simulink model "non_lin_dyn_model"  (R2024b)
settings: Solver=ode4  StartTime=0.0  StopTime=30  FixedStep=ST  RelTol=1e-3
values from neighbouring files (symbols this model uses):
  AOP = 2.75*pi/180    (= 0.0479965544298)    [parameters.m]
  AOPTR = 0    [parameters.m]
  ASLOPE = 6.28    [parameters.m]
  ASLOPETR = 6.28    [parameters.m]
  att_sp = 0    [FEL_RBFNN.m]    (also in results.m)
  Ax = 5.5*0.3048^2    (= 0.51096672)    [parameters.m]
  Ay = 156.1*0.3048^2    (= 14.502164544)    [parameters.m]
  Az = 84.7*0.3048^2    (= 7.868887488)    [parameters.m]
  B_inv = inv(B*B_dim)    [parameters.m]
  BLADES = 2    [parameters.m]
  BLADESTR = 2    [parameters.m]
  CD_mr = [0.009 0 0.3]    [parameters.m]
  CD_tr = [0.009 0 0.3]    [parameters.m]
  CHORD = 2.25*Ft_m    (= 0.6858)    [parameters.m]
  CHORDTR = 0.7*Ft_m    (= 0.21336)    [parameters.m]
  eta = 1    [FEL_RBFNN.m]
  f = [ 0; 0; Q_mr_trim/Izz]    [parameters.m]
  g = 9.81    [parameters.m]
  GAMMA = 5.216    [parameters.m]
  k = diag([3.7,5,10])    [FEL_RBFNN.m]
  k_ind = 1    [parameters.m]
  L_fus = [ -0.1 ... (first row only)    [parameters.m]
  L_mr = [  -0.1 ... (first row only)    [parameters.m]
  L_tr = [  -8.25 ... (first row only)    [parameters.m]
  lambda = diag([0.08,0.05,1.5])    [FEL_RBFNN.m]
  lat_cyc_range = [ -15 15 ]    [parameters.m]
  lon_cyc_range = [ -15 15 ]    [parameters.m]
  m = 8000*Lb_Kg    (= 3628.736)    [parameters.m]
  mr_coll_range = [ 7.5 25 ]    [parameters.m]
  NN_state = 1    [FEL_RBFNN.m]    (also in results.m)
  OMEGA = 314*(pi/30)    (= 32.8820031076)    [parameters.m]
  OMEGATR = 1608.5*(pi/30)    (= 168.44172611)    [parameters.m]
  pilot_trim = [-0.11603144404 0.198191531149 -0.14266835704 0.401015389998]    [hover_trim.mat]
  rho = 1.225    [parameters.m]
  ROTOR = 22*Ft_m    (= 6.7056)    [parameters.m]
  ROTORTR = 4.25*Ft_m    (= 1.2954)    [parameters.m]
  sigma = linspace(1.2,4.2,neurons)'    [FEL_RBFNN.m]
  ST = 0.01    [parameters.m]
  T_flap = 16/GAMMA/OMEGA    (= 0.0932876459059)    [parameters.m]
  THETT = -10*(pi/180)    (= -0.174532925199)    [parameters.m]
  THETTTR = 0*(pi/180)    (= 0)    [parameters.m]
  tr_coll_range = [ -20 20 ]    [parameters.m]
  vel_sp = 1    [FEL_RBFNN.m]    (also in results.m = 0)
  W0 = zeros(neurons,3)    [FEL_RBFNN.m]
  wind = 0    [FEL_RBFNN.m]    (also in results.m = 1)
  x0 = linspace(-1,1,neurons)'    [FEL_RBFNN.m]
  Xe_0 = [ 16404 0 -100 ]'*Ft_m    [parameters.m]
undefined symbols (not defined in the file or in its folder): rad, s
libraries: matrix_library x3, slpidlib x3, aerolibsim3d x2, sim3dlib x1, aerolibconvert2 x1, shared6dof x1, aerolibanimutils x1
(part 1 of 2)
settings Model: Creator=fra62  LastModifiedBy=fra62

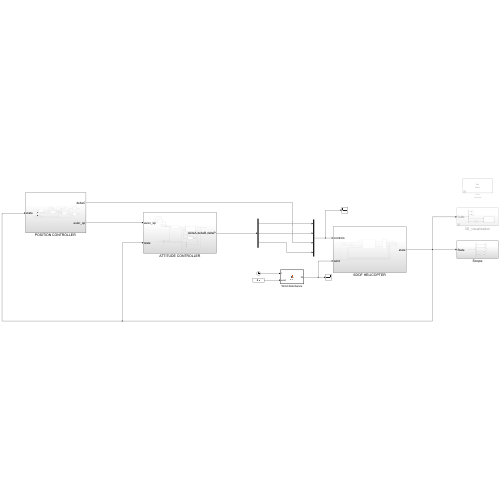
[thumbnail: Simulink's stored preview of the top-level diagram]
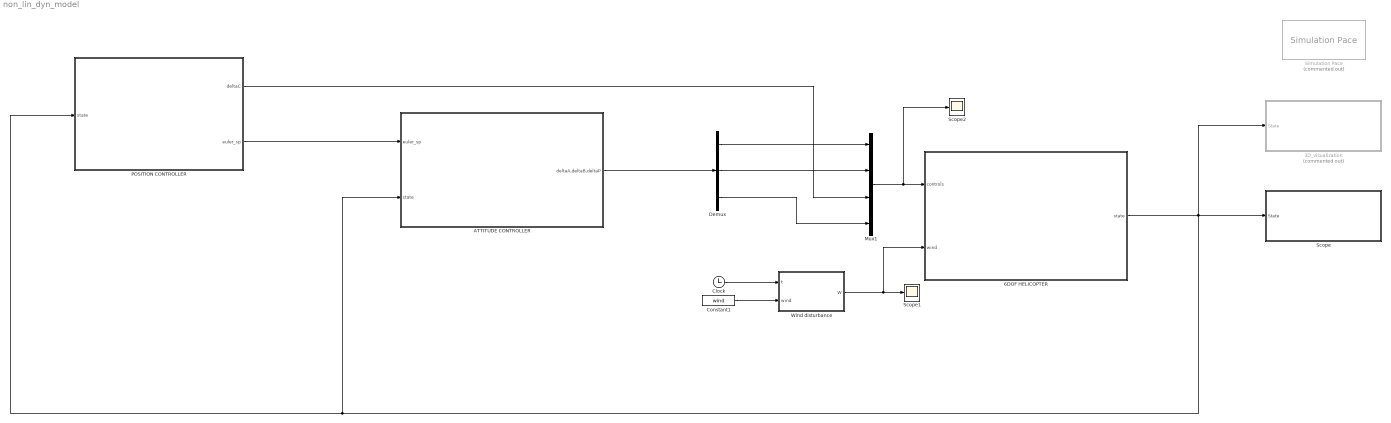
== system non_lin_dyn_model ==
  3D_visualization : Subsystem  Commented=on
  6DOF HELICOPTER : Subsystem
  ATTITUDE CONTROLLER : Subsystem
  Clock : Clock
  Constant1 : Constant  Value=wind
  Demux : Demux  Outputs=3
  Mux1 : Mux
  "POSITION CONTROLLER " : Subsystem
  Scope : Subsystem
  Scope1 : Scope
  Scope2 : Scope
  Simulation Pace : aerolibanimutils/Simulation Pace  Commented=on  SimulationPace=1  SleepMode=Auto  OutputPaceError=off  SampleTime=-1
  Wind disturbance : MATLAB Function  TreatAsAtomicUnit=on
  wires:
  6DOF HELICOPTER/1(state) -> "POSITION CONTROLLER "/1(state), ATTITUDE CONTROLLER/2(state), 3D_visualization/1(State), Scope/1(State)
  Demux/2 -> Mux1/2
  Demux/3 -> Mux1/4
  Demux/1 -> Mux1/1
  Mux1/1 -> Scope2/1, 6DOF HELICOPTER/1(controls)
  "POSITION CONTROLLER "/1(deltaC) -> Mux1/3
  ATTITUDE CONTROLLER/1(deltaA,deltaB,deltaP) -> Demux/1
  "POSITION CONTROLLER "/2(euler_sp) -> ATTITUDE CONTROLLER/1(euler_sp)
  Clock/1 -> Wind disturbance/1(t)
  Constant1/1 -> Wind disturbance/2(wind)
  Wind disturbance/1(W) -> Scope1/1, 6DOF HELICOPTER/2(wind)

== system non_lin_dyn_model/3D_visualization ==
  State : Inport
  Bus Selector : BusSelector  OutputSignals=Ve,omega,Xe,euler
  Reshape : Reshape
  Terminator : Terminator
  Terminator1 : Terminator
  UNREAL ENGINE 3D SCENE : Subsystem
  wires:
  Bus Selector/3 -> UNREAL ENGINE 3D SCENE/1(Xe)  "<Xe>"
  Bus Selector/4 -> Reshape/1  "<euler>"
  Bus Selector/2 -> Terminator1/1  "<omega>"
  State/1 -> Bus Selector/1
  Reshape/1 -> UNREAL ENGINE 3D SCENE/2(euler)
  Bus Selector/1 -> Terminator/1  "<Ve>"

== system non_lin_dyn_model/6DOF HELICOPTER ==
  controls : Inport
  wind : Inport  Port=2
  6DOF (Euler Angles) : shared6dof/6DOF (Euler Angles)  units=Metric (MKS)  mtype=Fixed  rep=Euler Angles  xme_0=Xe_0  Vm_0=V0  eul_0=euler0  pm_0=omega0  mass_0=m  mass_e=0.5  mass_f=2.0  inertia=inertia  inertia_e=eye(3)  inertia_f=2*eye(3)  k_quat=1.0  vre_flag=on  abi_flag=off  aMode=0  xme_statename=''  Vm_statename=''  eul_statename=''  quat_statename=''  pm_statename=''  mass_statename=''
  Add : Sum  Inputs=-+
  Bus Creator : BusCreator  Inputs=5
  HELICOPTER FORCES AND MOMENTS : Subsystem
  Matrix Multiply1 : Product  Multiplication=Matrix(*)
  Terminator1 : Terminator
  state : Outport
  wires:
  controls/1 -> HELICOPTER FORCES AND MOMENTS/1(controls)
  6DOF (Euler Angles)/8 -> Terminator1/1
  HELICOPTER FORCES AND MOMENTS/1(F_b) -> 6DOF (Euler Angles)/1
  6DOF (Euler Angles)/7 -> Bus Creator/5  "omega_dot"
  6DOF (Euler Angles)/4 -> HELICOPTER FORCES AND MOMENTS/2(Tbe), Matrix Multiply1/1
  6DOF (Euler Angles)/5 -> Add/2
  Add/1 -> HELICOPTER FORCES AND MOMENTS/3(TAS)
  6DOF (Euler Angles)/6 -> HELICOPTER FORCES AND MOMENTS/4(omega_b), Bus Creator/4  "omega"
  HELICOPTER FORCES AND MOMENTS/2(M_b) -> 6DOF (Euler Angles)/2
  6DOF (Euler Angles)/1 -> Bus Creator/1  "Ve"
  6DOF (Euler Angles)/2 -> Bus Creator/2  "Xe"
  6DOF (Euler Angles)/3 -> Bus Creator/3  "euler"
  Bus Creator/1 -> state/1
  Matrix Multiply1/1 -> Add/1
  wind/1 -> Matrix Multiply1/2

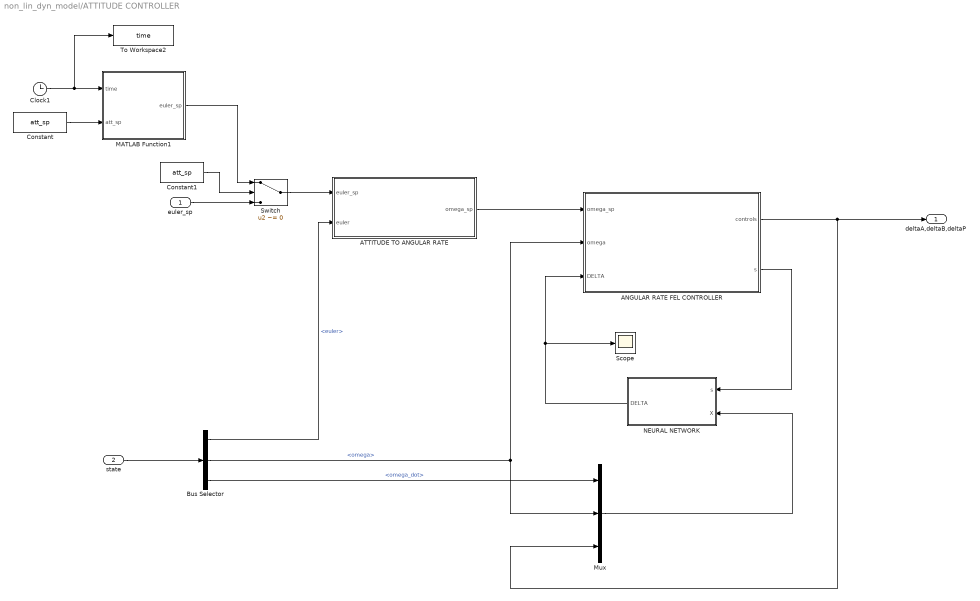
== system non_lin_dyn_model/ATTITUDE CONTROLLER ==
  euler_sp : Inport
  state : Inport  Port=2
  "ANGULAR RATE FEL CONTROLLER " : Subsystem
  ATTITUDE TO ANGULAR RATE : Subsystem
  Bus Selector : BusSelector  OutputSignals=euler,omega,omega_dot
  Clock1 : Clock
  Constant : Constant  Value=att_sp
  Constant1 : Constant  Value=att_sp
  MATLAB Function1 : MATLAB Function  TreatAsAtomicUnit=on
  Mux : Mux  Inputs=3
  "NEURAL NETWORK " : Subsystem
  Scope : Scope
  Switch : Switch  Criteria=u2 ~= 0  SaturateOnIntegerOverflow=off  InputSameDT=off
  To Workspace2 : ToWorkspace  VariableName=time  SampleTime=-1
  deltaA,deltaB,deltaP : Outport
  wires:
  Bus Selector/2 -> "ANGULAR RATE FEL CONTROLLER "/2(omega), Mux/2  "<omega>"
  Bus Selector/3 -> Mux/1  "<omega_dot>"
  state/1 -> Bus Selector/1
  "ANGULAR RATE FEL CONTROLLER "/1(controls) -> deltaA,deltaB,deltaP/1, Mux/3
  Switch/1 -> ATTITUDE TO ANGULAR RATE/1(euler_sp)
  ATTITUDE TO ANGULAR RATE/1(omega_sp) -> "ANGULAR RATE FEL CONTROLLER "/1(omega_sp)
  Mux/1 -> "NEURAL NETWORK "/2(X)
  "NEURAL NETWORK "/1(DELTA) -> "ANGULAR RATE FEL CONTROLLER "/3(DELTA), Scope/1
  Bus Selector/1 -> ATTITUDE TO ANGULAR RATE/2(euler)  "<euler>"
  "ANGULAR RATE FEL CONTROLLER "/2(s) -> "NEURAL NETWORK "/1(s)
  Constant/1 -> MATLAB Function1/2(att_sp)
  Clock1/1 -> To Workspace2/1, MATLAB Function1/1(time)
  Constant1/1 -> Switch/2
  euler_sp/1 -> Switch/3
  MATLAB Function1/1(euler_sp) -> Switch/1

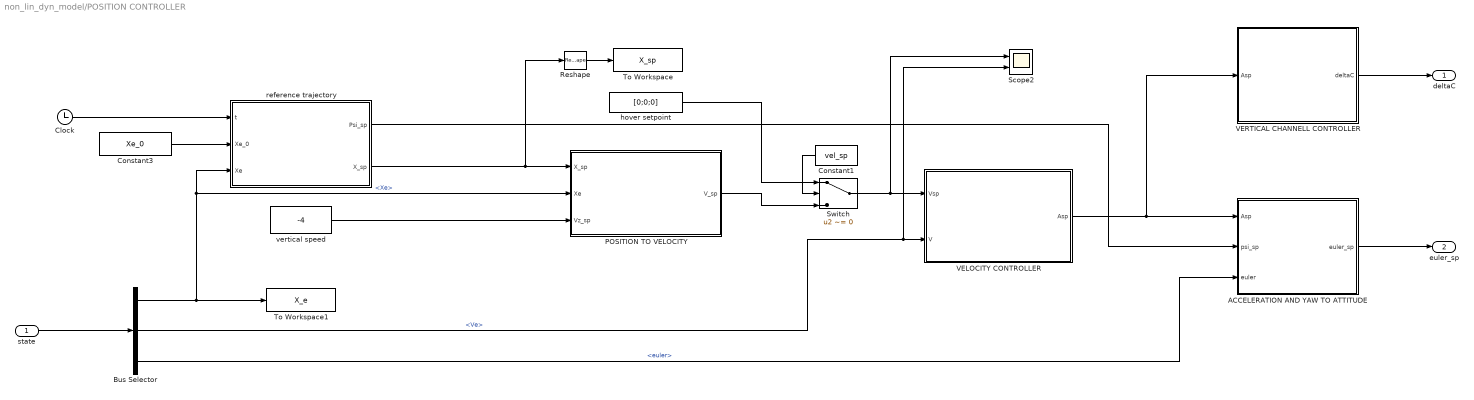
== system non_lin_dyn_model/POSITION CONTROLLER  ==
  state : Inport
  ACCELERATION AND YAW TO ATTITUDE : Subsystem
  Bus Selector : BusSelector  OutputSignals=Xe,Ve,euler
  Clock : Clock
  Constant1 : Constant  Value=vel_sp
  Constant3 : Constant  Value=Xe_0
  POSITION TO VELOCITY : Subsystem
  Reshape : Reshape
  Scope2 : Scope  NumInputPorts=2
  Switch : Switch  Criteria=u2 ~= 0  SaturateOnIntegerOverflow=off  InputSameDT=off
  To Workspace : ToWorkspace  VariableName=X_sp  SampleTime=-1
  To Workspace1 : ToWorkspace  VariableName=X_e  SampleTime=-1
  VELOCITY CONTROLLER : Subsystem
  VERTICAL CHANNELL CONTROLLER : Subsystem
  hover setpoint : Constant  Value=[0;0;0]
  reference trajectory : MATLAB Function  TreatAsAtomicUnit=on
  vertical speed : Constant  Value=-4
  deltaC : Outport
  euler_sp : Outport  Port=2
  wires:
  VERTICAL CHANNELL CONTROLLER/1(deltaC) -> deltaC/1
  Switch/1 -> Scope2/1, VELOCITY CONTROLLER/1(Vsp)
  reference trajectory/2(X_sp) -> Reshape/1, POSITION TO VELOCITY/1(X_sp)
  VELOCITY CONTROLLER/1(Asp) -> VERTICAL CHANNELL CONTROLLER/1(Asp), ACCELERATION AND YAW TO ATTITUDE/1(Asp)
  Bus Selector/2 -> VELOCITY CONTROLLER/2(V), Scope2/2  "<Ve>"
  Bus Selector/3 -> ACCELERATION AND YAW TO ATTITUDE/3(euler)  "<euler>"
  Bus Selector/1 -> To Workspace1/1, reference trajectory/3(Xe), POSITION TO VELOCITY/2(Xe)  "<Xe>"
  state/1 -> Bus Selector/1
  Constant3/1 -> reference trajectory/2(Xe_0)
  ACCELERATION AND YAW TO ATTITUDE/1(euler_sp) -> euler_sp/1
  Clock/1 -> reference trajectory/1(t)
  Reshape/1 -> To Workspace/1
  reference trajectory/1(Psi_sp) -> ACCELERATION AND YAW TO ATTITUDE/2(psi_sp)
  vertical speed/1 -> POSITION TO VELOCITY/3(Vz_sp)
  Constant1/1 -> Switch/2
  hover setpoint/1 -> Switch/1
  POSITION TO VELOCITY/1(V_sp) -> Switch/3

== system non_lin_dyn_model/Scope ==
  State : Inport
  Bus Selector : BusSelector  OutputSignals=Ve,omega,Xe,euler
  Gain : Gain  Gain=180/pi
  attitude : Scope
  position : Scope
  rates : Scope
  velocity : Scope
  wires:
  State/1 -> Bus Selector/1
  Gain/1 -> attitude/1
  Bus Selector/1 -> velocity/1  "<Ve>"
  Bus Selector/2 -> rates/1  "<omega>"
  Bus Selector/3 -> position/1  "<Xe>"
  Bus Selector/4 -> Gain/1  "<euler>"

== system non_lin_dyn_model/3D_visualization/UNREAL ENGINE 3D SCENE ==
  Xe : Inport
  euler : Inport  Port=2
  Constant : Constant  Value=OMEGA
  Constant1 : Constant  Value=100
  Simulation 3D Light Helicopter Pack : aerolibsim3d/Simulation 3D Light Helicopter Pack  Engine_T=off  Engine_R=off  Rotor1_T=off  Rotor1_R=on  Rotor2_T=off  Rotor2_R=on  Sensor1_T=off  Sensor1_R=off  Sensor2_T=off  Sensor2_R=off  GeoRadioButton=NED  AdjustForCesium=off  Heading0=90
  Simulation 3D Rotorcraft : aerolibsim3d/Simulation 3D Rotorcraft  Priority=-1  Mesh=Light helicopter  MeshPath=/MathWorksAerospaceContent/Vehicles/Rotorcraft/Helicopter/Mesh/SK_Helicopter.SK_Helicopter  MeshPathLight=/MathWorksAerospaceContent/Vehicles/Rotorcraft/LightHelicopter/Mesh/SK_LightHelicopter.SK_LightHelicopter  MeshPathMulti=/MathWorksAerospaceContent/Vehicles/Rotorcraft/Multirotor/Mesh/SK_Quadcopter.SK_Quadcopter  AircraftColor=Red  ActorName=helicopter  Translation=[Xe_0(1) Xe_0(2) Xe_0(3);zeros(5,3)]  Rotation=zeros(6, 3)  ScaleInputPort=Dialog  Scale=[1 1 1]  InitialScale=[1 1 1]  IsGHSensorEnabled=off  AreGHRaysVisible=off  IsOutputReshapeEnabled=off  GHRayLength=1524  GHBodyOffset=1.169  GHFrontTireRadius=0.196  GHLeftTireRadius=0.203  GHRightTireRadius=0.203  GHContactLocation1=[1.47 -1.04 1.169]  GHContactLocation2=[-1.24 -1.04 1.169]  GHContactLocation3=[-1.24 1.04 1.169]  GHContactLocation4=[1.47 1.04 1.169]  WoWSensorTolerance=0.05  LightsConfig=Automatic lights  LandingLightIntensity=300000  LandingLightConeAngle=15  LandingLightColor=[1 1 1]  HelicopterLeftLandingLightLocation=[0 0 0]  HelicopterLeftLandingLightOrientation=[0 0 0]  NoseLightIntensity=150000  NoseLightConeAngle=36  HelicopterNoseLightLocation=[0 0 0]  HelicopterNoseLightOrientation=[0 0 0]  NavLightIntensity=500  PositionLightIntensity=500  StrobeLightIntensity=5000  StrobeLightColor=[1 1 1]  StrobePeriod=1.5  StrobePulseWidth=6  BeaconLightIntensity=4000  BeaconLightColor=[1 0 0]  BeaconPeriod=1.5  BeaconPulseWidth=10  SampleTime=-1  ActorType=SimulinkVehicle  ID=C  aMode=0  ActorTag=helicopter
  Simulation 3D Scene Configuration1 : sim3dlib/Simulation 3D Scene Configuration  Priority=0  ProjectFormat=Default Scenes  SceneDesc=Airport  ProjectName=C:\Program Files\MATLAB\R2024b\toolbox\shared\sim3d_projects\automotive_project_windows\UE\WindowsNoEditor\VehicleSimulation.exe  ScenePath=/Game/Maps/HwStrght  EnableOpenDRIVE=off  vehTagList={'Custom';'Prouty example helicopter (medium size utility)';'Scene Origin';'SimulinkVehicle1';'helicopter'}  vehTag=helicopter  FreeCameraInitialTranslation=[-6, 0, 2]  FreeCameraDefaultInitialTranslation=[-6, 0, 2]  FreeCameraInitialRotation=[0, -15, 0]  FreeCameraDefaultInitialRotation=[0, -15, 0]  OpVisEn=off  Ts=.03  EnableWindow=on  EnableRemoteAccess=off  EnableWeather=off  SunAzimuth=90  SunAltitude=40.0  EnableGeospatialSun=off  Latitude=0  Longitude=0  Date=2023-01-01  Time=10:30:00  GeoTimeZone=-5.0  SunDaylightSaving=off  wind=1  clouds=10  EnableVolumetricClouds=off  CloudCoverage=0  CloudAltitude=6  fog=0  rain=0  RaindropsEffect=off  SnowDensity=0  EnableGeospatial=off  UseTrueOrigin=off  OriginHeight=200  OriginLatitude=40.744652  OriginLongitude=-73.988864  MapStyle=Aerial  AdditionalAssetIDs=[]  UseAdvancedSunSky=off  SolarTime=11  TimeZone=-5  Day=21  Month=9  Year=2022  UseDaylightSavingTime=on  DSTStartDay=10  DSTStartMonth=3  DSTEndDay=3  DSTEndMonth=11  DSTSwitchHour=2  sensorTag=MainCamera2  sensorId=2  sensorName=MainCamera2  mountLoc=Origin  offsetFlag=off  tmountOffset=[0, 0, 0]  rmountOffset=[0, 0, 0]  HorizontalResolution=1280  VerticalResolution=720  HorizontalFOV=60  mountPoint=[0 0 0]  mountOrientation=[0 0 0]  aMode=0  ID=2  GeoTrigger=Inactive
      settings: LibrarySourceBlock=aerolibsim3d/Simulation 3D Scene Configuration
  Subsystem : Subsystem
  wires:
  Constant1/1 -> Subsystem/2(SpeedT)
  Constant/1 -> Subsystem/1(SpeedM)
  Subsystem/2(Position Blade 2) -> Simulation 3D Light Helicopter Pack/4
  Subsystem/1(Position Blade1) -> Simulation 3D Light Helicopter Pack/3
  Simulation 3D Light Helicopter Pack/1 -> Simulation 3D Rotorcraft/1
  Simulation 3D Light Helicopter Pack/2 -> Simulation 3D Rotorcraft/2
  euler/1 -> Simulation 3D Light Helicopter Pack/2
  Xe/1 -> Simulation 3D Light Helicopter Pack/1

== system non_lin_dyn_model/6DOF HELICOPTER/HELICOPTER FORCES AND MOMENTS ==
  controls : Inport
  Tbe : Inport  Port=2
  TAS : Inport  Port=3
  omega_b : Inport  Port=4
  CG FORCES : Sum  Inputs=++++
  CG MOMENTS : Sum  Inputs=+++
  CONTROL MIXER : Subsystem
  Demux1 : Demux
  FUSELAGE : Subsystem
  GRAVITY : Subsystem
  MAIN ROTOR : Subsystem
  TAIL ROTOR : Subsystem
  F_b : Outport
  M_b : Outport  Port=2
  wires:
  CG MOMENTS/1 -> M_b/1
  CONTROL MIXER/4(TR COLLECTIVE) -> TAIL ROTOR/1(theta0_tr)
  MAIN ROTOR/1(F_mr) -> CG FORCES/2
  TAIL ROTOR/2(M_tr) -> CG MOMENTS/2
  FUSELAGE/1(F_fus) -> CG FORCES/4
  CONTROL MIXER/1(A1s) -> MAIN ROTOR/3(A1s)
  MAIN ROTOR/2(M_mr) -> CG MOMENTS/1
  omega_b/1 -> MAIN ROTOR/2(omega)
  TAS/1 -> MAIN ROTOR/1(TAS), FUSELAGE/1(TAS)
  CG FORCES/1 -> F_b/1
  TAIL ROTOR/1(F_tr) -> CG FORCES/3
  FUSELAGE/2(M_fus) -> CG MOMENTS/3
  CONTROL MIXER/3(MR COLLECTIVE) -> MAIN ROTOR/5(theta0_mr)
  CONTROL MIXER/2(B1s) -> MAIN ROTOR/4(B1s)
  Tbe/1 -> GRAVITY/1(Tbe)
  GRAVITY/1(F_g) -> CG FORCES/1
  Demux1/3 -> CONTROL MIXER/3(deltaC)  "collective"
  Demux1/2 -> CONTROL MIXER/2(deltaB)  "longitudinal cyc"
  Demux1/4 -> CONTROL MIXER/4(deltaP)  "pedals"
  Demux1/1 -> CONTROL MIXER/1(deltaA)  "lateral cyc"
  controls/1 -> Demux1/1

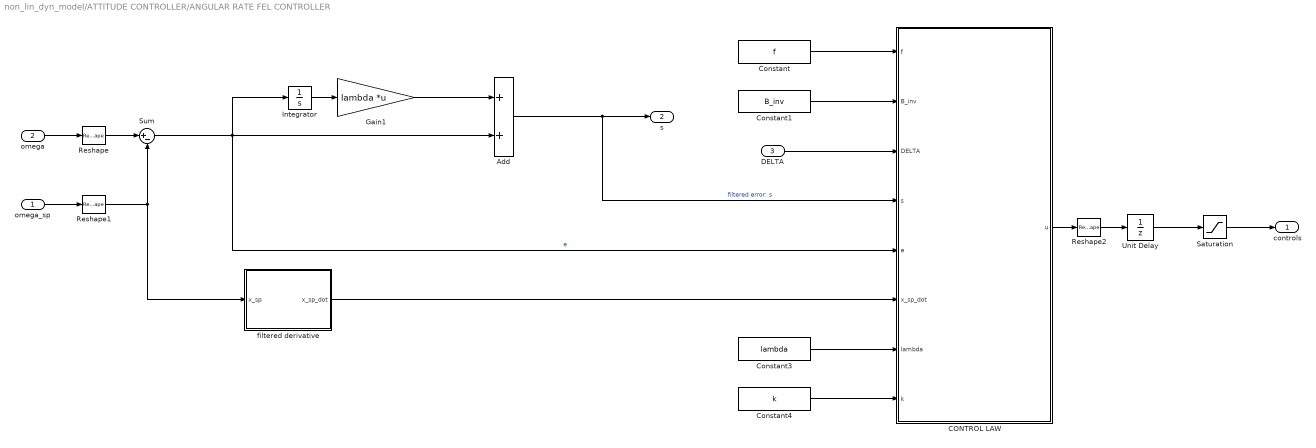
== system non_lin_dyn_model/ATTITUDE CONTROLLER/ANGULAR RATE FEL CONTROLLER  ==
  omega_sp : Inport
  omega : Inport  Port=2
  DELTA : Inport  Port=3
  Add : Sum
  CONTROL LAW : MATLAB Function  TreatAsAtomicUnit=on
  Constant : Constant  Value=f
  Constant1 : Constant  Value=B_inv
  Constant3 : Constant  Value=lambda
  Constant4 : Constant  Value=k
  Gain1 : Gain  Gain=lambda  Multiplication=Matrix(K*u) (u vector)
  Integrator : Integrator
  Reshape : Reshape  OutputDimensionality=Column vector (2-D)
  Reshape1 : Reshape  OutputDimensionality=Column vector (2-D)
  Reshape2 : Reshape  OutputDimensionality=Column vector (2-D)
  Saturation : Saturate  UpperLimit=1  LowerLimit=-1
  Sum : Sum  Inputs=|+-
  Unit Delay : UnitDelay  SampleTime=-1  HasFrameUpgradeWarning=on
  filtered derivative : Subsystem
  controls : Outport
  s : Outport  Port=2
  wires:
  CONTROL LAW/1(u) -> Reshape2/1
  Saturation/1 -> controls/1
  Constant/1 -> CONTROL LAW/1(f)
  Constant1/1 -> CONTROL LAW/2(B_inv)
  DELTA/1 -> CONTROL LAW/3(DELTA)
  Constant3/1 -> CONTROL LAW/7(lambda)
  Constant4/1 -> CONTROL LAW/8(k)
  omega_sp/1 -> Reshape1/1
  omega/1 -> Reshape/1
  Reshape1/1 -> filtered derivative/1(x_sp), Sum/2
  filtered derivative/1(x_sp_dot) -> CONTROL LAW/6(x_sp_dot)
  Sum/1 -> Integrator/1, Add/2, CONTROL LAW/5(e)  "e"
  Add/1 -> s/1, CONTROL LAW/4(s)  "filtered error: s"
  Gain1/1 -> Add/1
  Integrator/1 -> Gain1/1
  Reshape/1 -> Sum/1
  Reshape2/1 -> Unit Delay/1
  Unit Delay/1 -> Saturation/1

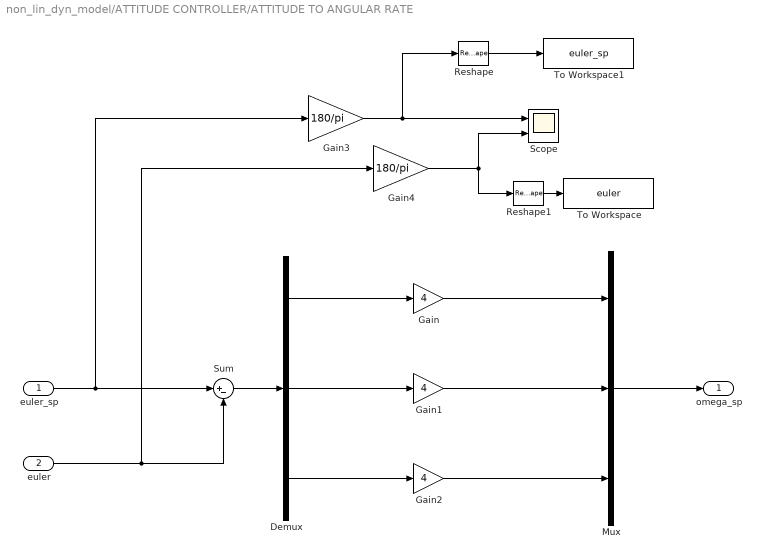
== system non_lin_dyn_model/ATTITUDE CONTROLLER/ATTITUDE TO ANGULAR RATE ==
  euler_sp : Inport
  euler : Inport  Port=2
  Demux : Demux  Outputs=3
  Gain : Gain  Gain=4
  Gain1 : Gain  Gain=4
  Gain2 : Gain  Gain=4
  Gain3 : Gain  Gain=180/pi
  Gain4 : Gain  Gain=180/pi
  Mux : Mux  Inputs=3
  Reshape : Reshape  OutputDimensionality=Column vector (2-D)
  Reshape1 : Reshape  OutputDimensionality=Column vector (2-D)
  Scope : Scope  NumInputPorts=2
  Sum : Sum  Inputs=|+-
  To Workspace : ToWorkspace  VariableName=euler  SampleTime=-1
  To Workspace1 : ToWorkspace  VariableName=euler_sp  SampleTime=-1
  omega_sp : Outport
  wires:
  Gain2/1 -> Mux/3
  euler/1 -> Gain4/1, Sum/2
  Mux/1 -> omega_sp/1
  Demux/3 -> Gain2/1
  Demux/2 -> Gain1/1
  Gain/1 -> Mux/1
  euler_sp/1 -> Gain3/1, Sum/1
  Demux/1 -> Gain/1
  Sum/1 -> Demux/1
  Gain1/1 -> Mux/2
  Gain3/1 -> Reshape/1, Scope/1
  Gain4/1 -> Reshape1/1, Scope/2
  Reshape/1 -> To Workspace1/1
  Reshape1/1 -> To Workspace/1

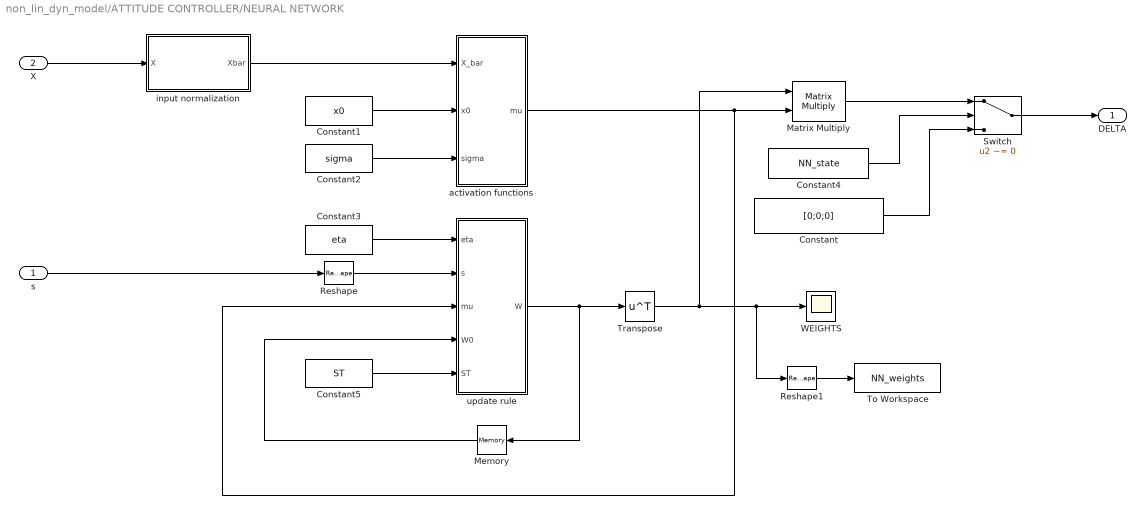
== system non_lin_dyn_model/ATTITUDE CONTROLLER/NEURAL NETWORK  ==
  s : Inport
  X : Inport  Port=2
  Constant : Constant  Value=[0;0;0]
  Constant1 : Constant  Value=x0
  Constant2 : Constant  Value=sigma
  Constant3 : Constant  Value=eta
  Constant4 : Constant  Value=NN_state
  Constant5 : Constant  Value=ST
  Matrix Multiply : Product  Multiplication=Matrix(*)
  Memory : Memory  InitialCondition=W0
  Reshape : Reshape  OutputDimensionality=Column vector (2-D)
  Reshape1 : Reshape  OutputDimensionality=Column vector (2-D)
  Switch : Switch  Criteria=u2 ~= 0  SaturateOnIntegerOverflow=off  InputSameDT=off
  To Workspace : ToWorkspace  VariableName=NN_weights  SampleTime=-1
  Transpose : Math  Operator=transpose
  WEIGHTS : Scope
  activation functions : MATLAB Function  TreatAsAtomicUnit=on
  input normalization : MATLAB Function  TreatAsAtomicUnit=on
  update rule : MATLAB Function  TreatAsAtomicUnit=on
  DELTA : Outport
  wires:
  Constant2/1 -> activation functions/3(sigma)
  Constant3/1 -> update rule/1(eta)
  s/1 -> Reshape/1
  X/1 -> input normalization/1(X)
  activation functions/1(mu) -> Matrix Multiply/2, update rule/3(mu)
  Constant1/1 -> activation functions/2(x0)
  input normalization/1(Xbar) -> activation functions/1(X_bar)
  Reshape/1 -> update rule/2(s)
  update rule/1(W) -> Transpose/1, Memory/1
  Transpose/1 -> Matrix Multiply/1, Reshape1/1, WEIGHTS/1
  Switch/1 -> DELTA/1
  Matrix Multiply/1 -> Switch/1
  Constant/1 -> Switch/3
  Constant4/1 -> Switch/2
  Memory/1 -> update rule/4(W0)
  Constant5/1 -> update rule/5(ST)
  Reshape1/1 -> To Workspace/1

== system non_lin_dyn_model/POSITION CONTROLLER /ACCELERATION AND YAW TO ATTITUDE ==
  Asp : Inport
  psi_sp : Inport  Port=2
  euler : Inport  Port=3
  Constant : Constant  Value=9.81
  MATLAB Function : MATLAB Function  TreatAsAtomicUnit=on
  Mux : Mux  Inputs=3
  Reshape : Reshape  OutputDimensionality=Column vector (2-D)
  Selector : Selector  InputPortWidth=3  IndexOptions=Index vector (dialog)  Indices=3  OutputSizes=1
  Transfer Fcn : TransferFcn  Numerator=[1/0.1]  Denominator=[1 1/0.1]
  euler_sp : Outport
  wires:
  MATLAB Function/2(theta_sp) -> Transfer Fcn/1
  Asp/1 -> MATLAB Function/1(Asp)
  Constant/1 -> MATLAB Function/2(g0)
  Mux/1 -> Reshape/1
  psi_sp/1 -> Mux/3
  Reshape/1 -> euler_sp/1
  euler/1 -> Selector/1
  Selector/1 -> MATLAB Function/3(psi)
  MATLAB Function/1(phi_sp) -> Mux/1
  Transfer Fcn/1 -> Mux/2

== system non_lin_dyn_model/POSITION CONTROLLER /POSITION TO VELOCITY ==
  X_sp : Inport
  Xe : Inport  Port=2
  Vz_sp : Inport  Port=3
  Gain : Gain
  Gain1 : Gain
  Mux2 : Mux  Inputs=3
  Selector1 : Selector  InputPortWidth=3  IndexOptions=Index vector (dialog)  Indices=1  OutputSizes=1
  Selector2 : Selector  InputPortWidth=3  IndexOptions=Index vector (dialog)  Indices=2  OutputSizes=1
  Sum : Sum  Inputs=|+-
  V_sp : Outport
  wires:
  Gain/1 -> Mux2/1
  Selector1/1 -> Gain/1
  Sum/1 -> Selector2/1, Selector1/1
  Mux2/1 -> V_sp/1
  Xe/1 -> Sum/2
  Selector2/1 -> Gain1/1
  X_sp/1 -> Sum/1
  Gain1/1 -> Mux2/2
  Vz_sp/1 -> Mux2/3

== system non_lin_dyn_model/POSITION CONTROLLER /VELOCITY CONTROLLER ==
  Vsp : Inport
  V : Inport  Port=2
  Mux : Mux  Inputs=3
  PID Controller1 : slpidlib/PID Controller  Controller=PID  Form=Parallel  TimeDomain=Continuous-time  UseExternalTs=off  SampleTime=-1  IntegratorMethod=Forward Euler  FilterMethod=Forward Euler  ControllerParametersSource=internal  P=2  I=0.5  UseKiTs=off  D=0  UseExternalDerivativeSource=off  N=100  UseFilter=on  TunerSelectOption=Transfer Function Based (PID Tuner App)  InitialConditionSource=internal  InitialConditionForIntegrator=0  InitialConditionForFilter=0  DifferentiatorICPrevScaledInput=0  ExternalReset=none  TrackingMode=off  Kt=1  LimitOutput=on  SatLimitsSource=internal  UpperSaturationLimit=9.81  LowerSaturationLimit=-9.81  LinearizeAsGain=on  AntiWindupMode=none  Kb=1  LimitIntegrator=on  UpperIntegratorSaturationLimit=9.81  LowerIntegratorSaturationLimit=-9.81  POutMin=[]  POutMax=[]  IOutMin=[]  IOutMax=[]  DOutMin=[]  DOutMax=[]  NOutMin=[]  NOutMax=[]  SumOutMin=[]  SumOutMax=[]  SaturationOutMin=[]  SaturationOutMax=[]  PParamMin=[]  PParamMax=[]  IParamMin=[]  IParamMax=[]  DParamMin=[]  DParamMax=[]  NParamMin=[]  NParamMax=[]  KbParamMin=[]  KbParamMax=[]  KtParamMin=[]  KtParamMax=[]  KbOutMin=[]  KbOutMax=[]  KtOutMin=[]  KtOutMax=[]  IntegratorOutMin=[]  IntegratorOutMax=[]  FilterOutMin=[]  FilterOutMax=[]  SumI1OutMin=[]  SumI1OutMax=[]  SumI2OutMin=[]  SumI2OutMax=[]  SumI3OutMin=[]  SumI3OutMax=[]  SumI4OutMin=[]  SumI4OutMax=[]  SumDOutMin=[]  SumDOutMax=[]  DifferentiatorOutMin=[]  DifferentiatorOutMax=[]  FilterDiffOutCoefMin=[]  FilterDiffOutCoefMax=[]  ReciprocalOutMin=[]  ReciprocalOutMax=[]  SumDenOutMin=[]  SumDenOutMax=[]  SumNumOutMin=[]  SumNumOutMax=[]  DivideOutMin=[]  DivideOutMax=[]  UdiffTsProdOutMin=[]  UdiffTsProdOutMax=[]  NTsProdOutMin=[]  NTsProdOutMax=[]  UintegralTsProdOutMin=[]  UintegralTsProdOutMax=[]  UngainTsProdOutMin=[]  UngainTsProdOutMax=[]  ClampingZeroOutDataTypeStr=Inherit: Inherit via back propagation  ClampingZeroOutMin=[]  ClampingZeroOutMax=[]  FilterDenConstantOutDataTypeStr=Inherit: Inherit via back propagation  FilterDenConstantOutMin=[]  FilterDenConstantOutMax=[]  PCopyOutDataTypeStr=Inherit: Inherit via back propagation  PCopyOutMin=[]  PCopyOutMax=[]  NCopyOutDataTypeStr=Inherit: Inherit via back propagation  NCopyOutMin=[]  NCopyOutMax=[]  IntegratorContinuousStateAttributes=''  IntegratorStateMustResolveToSignalObject=off  IntegratorRTWStateStorageClass=Auto  FilterContinuousStateAttributes=''  FilterStateMustResolveToSignalObject=off  FilterRTWStateStorageClass=Auto  ParallelPVariant=InternalParameters  IdealPVariant=Disabled  IVariant=InternalParameters  DVariant=InternalParameters  IntegratorVariant=Continuous  SatVariant=Enabled  AWVariant=Passthrough  PCopyVariant=Disabled  TRVariant=Disabled  FdbkBlocksVariant=Forward  IdealPFdbkVariant=Disabled  SatFdbkVariant=Disabled  DerivativeFilterVariant=ContFilter  NVariant=InternalParameters  NCopyVariant=Disabled  FilterICVariant=InternalICsFilter  IntegratorICVariant=InternalICs  ExternalResetVariant=Disabled  TRSumVariant=Passthrough  SumFdbkVariant=Disabled  SumVariant=Sum_PID  TsampFilterVariant=InternalTs  TsampNgainVariant=Passthrough  TsampIntegralVariant=Disabled_SignalSpec  ExternalSaturationOutDataTypeStr=Inherit: Same as second input  DerivativeSourceVariant=ErrorSignal  PreIntVariant=InternalPreInt
  PID Controller2 : slpidlib/PID Controller  Controller=PID  Form=Parallel  TimeDomain=Continuous-time  UseExternalTs=off  SampleTime=-1  IntegratorMethod=Forward Euler  FilterMethod=Forward Euler  ControllerParametersSource=internal  P=1.4  I=0.6  UseKiTs=off  D=0.25  UseExternalDerivativeSource=off  N=100  UseFilter=on  TunerSelectOption=Transfer Function Based (PID Tuner App)  InitialConditionSource=internal  InitialConditionForIntegrator=0  InitialConditionForFilter=0  DifferentiatorICPrevScaledInput=0  ExternalReset=none  TrackingMode=off  Kt=1  LimitOutput=on  SatLimitsSource=internal  UpperSaturationLimit=9.81  LowerSaturationLimit=-9.81  LinearizeAsGain=on  AntiWindupMode=none  Kb=1  LimitIntegrator=on  UpperIntegratorSaturationLimit=9.81  LowerIntegratorSaturationLimit=-9.81  POutMin=[]  POutMax=[]  IOutMin=[]  IOutMax=[]  DOutMin=[]  DOutMax=[]  NOutMin=[]  NOutMax=[]  SumOutMin=[]  SumOutMax=[]  SaturationOutMin=[]  SaturationOutMax=[]  PParamMin=[]  PParamMax=[]  IParamMin=[]  IParamMax=[]  DParamMin=[]  DParamMax=[]  NParamMin=[]  NParamMax=[]  KbParamMin=[]  KbParamMax=[]  KtParamMin=[]  KtParamMax=[]  KbOutMin=[]  KbOutMax=[]  KtOutMin=[]  KtOutMax=[]  IntegratorOutMin=[]  IntegratorOutMax=[]  FilterOutMin=[]  FilterOutMax=[]  SumI1OutMin=[]  SumI1OutMax=[]  SumI2OutMin=[]  SumI2OutMax=[]  SumI3OutMin=[]  SumI3OutMax=[]  SumI4OutMin=[]  SumI4OutMax=[]  SumDOutMin=[]  SumDOutMax=[]  DifferentiatorOutMin=[]  DifferentiatorOutMax=[]  FilterDiffOutCoefMin=[]  FilterDiffOutCoefMax=[]  ReciprocalOutMin=[]  ReciprocalOutMax=[]  SumDenOutMin=[]  SumDenOutMax=[]  SumNumOutMin=[]  SumNumOutMax=[]  DivideOutMin=[]  DivideOutMax=[]  UdiffTsProdOutMin=[]  UdiffTsProdOutMax=[]  NTsProdOutMin=[]  NTsProdOutMax=[]  UintegralTsProdOutMin=[]  UintegralTsProdOutMax=[]  UngainTsProdOutMin=[]  UngainTsProdOutMax=[]  ClampingZeroOutDataTypeStr=Inherit: Inherit via back propagation  ClampingZeroOutMin=[]  ClampingZeroOutMax=[]  FilterDenConstantOutDataTypeStr=Inherit: Inherit via back propagation  FilterDenConstantOutMin=[]  FilterDenConstantOutMax=[]  PCopyOutDataTypeStr=Inherit: Inherit via back propagation  PCopyOutMin=[]  PCopyOutMax=[]  NCopyOutDataTypeStr=Inherit: Inherit via back propagation  NCopyOutMin=[]  NCopyOutMax=[]  IntegratorContinuousStateAttributes=''  IntegratorStateMustResolveToSignalObject=off  IntegratorRTWStateStorageClass=Auto  FilterContinuousStateAttributes=''  FilterStateMustResolveToSignalObject=off  FilterRTWStateStorageClass=Auto  ParallelPVariant=InternalParameters  IdealPVariant=Disabled  IVariant=InternalParameters  DVariant=InternalParameters  IntegratorVariant=Continuous  SatVariant=Enabled  AWVariant=Passthrough  PCopyVariant=Disabled  TRVariant=Disabled  FdbkBlocksVariant=Forward  IdealPFdbkVariant=Disabled  SatFdbkVariant=Disabled  DerivativeFilterVariant=ContFilter  NVariant=InternalParameters  NCopyVariant=Disabled  FilterICVariant=InternalICsFilter  IntegratorICVariant=InternalICs  ExternalResetVariant=Disabled  TRSumVariant=Passthrough  SumFdbkVariant=Disabled  SumVariant=Sum_PID  TsampFilterVariant=InternalTs  TsampNgainVariant=Passthrough  TsampIntegralVariant=Disabled_SignalSpec  ExternalSaturationOutDataTypeStr=Inherit: Same as second input  DerivativeSourceVariant=ErrorSignal  PreIntVariant=InternalPreInt
  PID Controller4 : slpidlib/PID Controller  Controller=PID  Form=Parallel  TimeDomain=Continuous-time  UseExternalTs=off  SampleTime=-1  IntegratorMethod=Forward Euler  FilterMethod=Forward Euler  ControllerParametersSource=internal  P=1.4  I=0.6  UseKiTs=off  D=0.25  UseExternalDerivativeSource=off  N=100  UseFilter=on  TunerSelectOption=Transfer Function Based (PID Tuner App)  InitialConditionSource=internal  InitialConditionForIntegrator=0  InitialConditionForFilter=0  DifferentiatorICPrevScaledInput=0  ExternalReset=none  TrackingMode=off  Kt=1  LimitOutput=on  SatLimitsSource=internal  UpperSaturationLimit=9.81  LowerSaturationLimit=-9.81  LinearizeAsGain=on  AntiWindupMode=none  Kb=1  LimitIntegrator=on  UpperIntegratorSaturationLimit=9.81  LowerIntegratorSaturationLimit=-9.81  POutMin=[]  POutMax=[]  IOutMin=[]  IOutMax=[]  DOutMin=[]  DOutMax=[]  NOutMin=[]  NOutMax=[]  SumOutMin=[]  SumOutMax=[]  SaturationOutMin=[]  SaturationOutMax=[]  PParamMin=[]  PParamMax=[]  IParamMin=[]  IParamMax=[]  DParamMin=[]  DParamMax=[]  NParamMin=[]  NParamMax=[]  KbParamMin=[]  KbParamMax=[]  KtParamMin=[]  KtParamMax=[]  KbOutMin=[]  KbOutMax=[]  KtOutMin=[]  KtOutMax=[]  IntegratorOutMin=[]  IntegratorOutMax=[]  FilterOutMin=[]  FilterOutMax=[]  SumI1OutMin=[]  SumI1OutMax=[]  SumI2OutMin=[]  SumI2OutMax=[]  SumI3OutMin=[]  SumI3OutMax=[]  SumI4OutMin=[]  SumI4OutMax=[]  SumDOutMin=[]  SumDOutMax=[]  DifferentiatorOutMin=[]  DifferentiatorOutMax=[]  FilterDiffOutCoefMin=[]  FilterDiffOutCoefMax=[]  ReciprocalOutMin=[]  ReciprocalOutMax=[]  SumDenOutMin=[]  SumDenOutMax=[]  SumNumOutMin=[]  SumNumOutMax=[]  DivideOutMin=[]  DivideOutMax=[]  UdiffTsProdOutMin=[]  UdiffTsProdOutMax=[]  NTsProdOutMin=[]  NTsProdOutMax=[]  UintegralTsProdOutMin=[]  UintegralTsProdOutMax=[]  UngainTsProdOutMin=[]  UngainTsProdOutMax=[]  ClampingZeroOutDataTypeStr=Inherit: Inherit via back propagation  ClampingZeroOutMin=[]  ClampingZeroOutMax=[]  FilterDenConstantOutDataTypeStr=Inherit: Inherit via back propagation  FilterDenConstantOutMin=[]  FilterDenConstantOutMax=[]  PCopyOutDataTypeStr=Inherit: Inherit via back propagation  PCopyOutMin=[]  PCopyOutMax=[]  NCopyOutDataTypeStr=Inherit: Inherit via back propagation  NCopyOutMin=[]  NCopyOutMax=[]  IntegratorContinuousStateAttributes=''  IntegratorStateMustResolveToSignalObject=off  IntegratorRTWStateStorageClass=Auto  FilterContinuousStateAttributes=''  FilterStateMustResolveToSignalObject=off  FilterRTWStateStorageClass=Auto  ParallelPVariant=InternalParameters  IdealPVariant=Disabled  IVariant=InternalParameters  DVariant=InternalParameters  IntegratorVariant=Continuous  SatVariant=Enabled  AWVariant=Passthrough  PCopyVariant=Disabled  TRVariant=Disabled  FdbkBlocksVariant=Forward  IdealPFdbkVariant=Disabled  SatFdbkVariant=Disabled  DerivativeFilterVariant=ContFilter  NVariant=InternalParameters  NCopyVariant=Disabled  FilterICVariant=InternalICsFilter  IntegratorICVariant=InternalICs  ExternalResetVariant=Disabled  TRSumVariant=Passthrough  SumFdbkVariant=Disabled  SumVariant=Sum_PID  TsampFilterVariant=InternalTs  TsampNgainVariant=Passthrough  TsampIntegralVariant=Disabled_SignalSpec  ExternalSaturationOutDataTypeStr=Inherit: Same as second input  DerivativeSourceVariant=ErrorSignal  PreIntVariant=InternalPreInt
  Reshape : Reshape  OutputDimensionality=Column vector (2-D)
  Selector : Selector  InputPortWidth=3  IndexOptions=Index vector (dialog)  Indices=1  OutputSizes=1
  Selector1 : Selector  InputPortWidth=3  IndexOptions=Index vector (dialog)  Indices=2  OutputSizes=1
  Selector2 : Selector  InputPortWidth=3  IndexOptions=Index vector (dialog)  Indices=3  OutputSizes=1
  Sum : Sum  Inputs=|+-
  Asp : Outport
  wires:
  Mux/1 -> Reshape/1
  Vsp/1 -> Sum/1
  V/1 -> Sum/2
  Selector/1 -> PID Controller2/1
  Sum/1 -> Selector2/1, Selector1/1, Selector/1
  Selector1/1 -> PID Controller4/1
  Selector2/1 -> PID Controller1/1
  PID Controller4/1 -> Mux/2
  PID Controller2/1 -> Mux/1
  PID Controller1/1 -> Mux/3
  Reshape/1 -> Asp/1

== system non_lin_dyn_model/POSITION CONTROLLER /VERTICAL CHANNELL CONTROLLER ==
  Asp : Inport
  Constant : Constant  Value=9.81
  MATLAB Function : MATLAB Function  TreatAsAtomicUnit=on
  Saturation : Saturate  UpperLimit=1  LowerLimit=-1
  Selector : Selector  InputPortWidth=3  IndexOptions=Index vector (dialog)  Indices=3  OutputSizes=1
  Sum : Sum  Inputs=|++
  hover trim value of collective : Constant  Value=pilot_trim(3)
  deltaC : Outport
  wires:
  Constant/1 -> MATLAB Function/2(g0)
  Asp/1 -> Selector/1
  MATLAB Function/1(delta_vert) -> Sum/1
  Sum/1 -> Saturation/1
  hover trim value of collective/1 -> Sum/2
  Saturation/1 -> deltaC/1
  Selector/1 -> MATLAB Function/1(Asp_z)

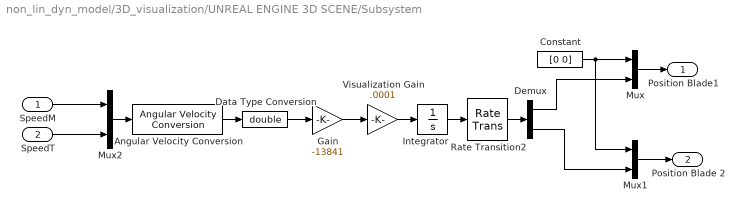
== system non_lin_dyn_model/3D_visualization/UNREAL ENGINE 3D SCENE/Subsystem ==
  SpeedM : Inport
  SpeedT : Inport  Port=2
  Angular Velocity Conversion : aerolibconvert2/Angular Velocity Conversion  IU=rad/s  OU=rpm
  Constant : Constant  Value=[0 0]  VectorParams1D=off
  Data Type Conversion : DataTypeConversion  OutDataTypeStr=double  SaturateOnIntegerOverflow=off  RndMeth=Floor
  Demux : Demux  Outputs=2
  Gain : Gain  Gain=-13841
  Integrator : Integrator  InitialCondition="[.1  .1]"  WrapState=on  WrappedStateUpperValue=2*pi  WrappedStateLowerValue=-2*pi
  Mux : Mux  Inputs=2
  Mux1 : Mux  Inputs=2
  Mux2 : Mux  Inputs=2
  Rate Transition2 : RateTransition
  Visualization Gain : Gain  Gain=.0001
  Position Blade1 : Outport  VectorParamsAs1DForOutWhenUnconnected=off
  Position Blade 2 : Outport  Port=2  VectorParamsAs1DForOutWhenUnconnected=off
  wires:
  Demux/2 -> Mux1/2
  Visualization Gain/1 -> Integrator/1
  Constant/1 -> Mux1/1, Mux/1
  Mux1/1 -> Position Blade 2/1
  Data Type Conversion/1 -> Gain/1
  Integrator/1 -> Rate Transition2/1
  Mux/1 -> Position Blade1/1
  Gain/1 -> Visualization Gain/1
  Demux/1 -> Mux/2
  Mux2/1 -> Angular Velocity Conversion/1
  Rate Transition2/1 -> Demux/1
  SpeedM/1 -> Mux2/1
  SpeedT/1 -> Mux2/2
  Angular Velocity Conversion/1 -> Data Type Conversion/1

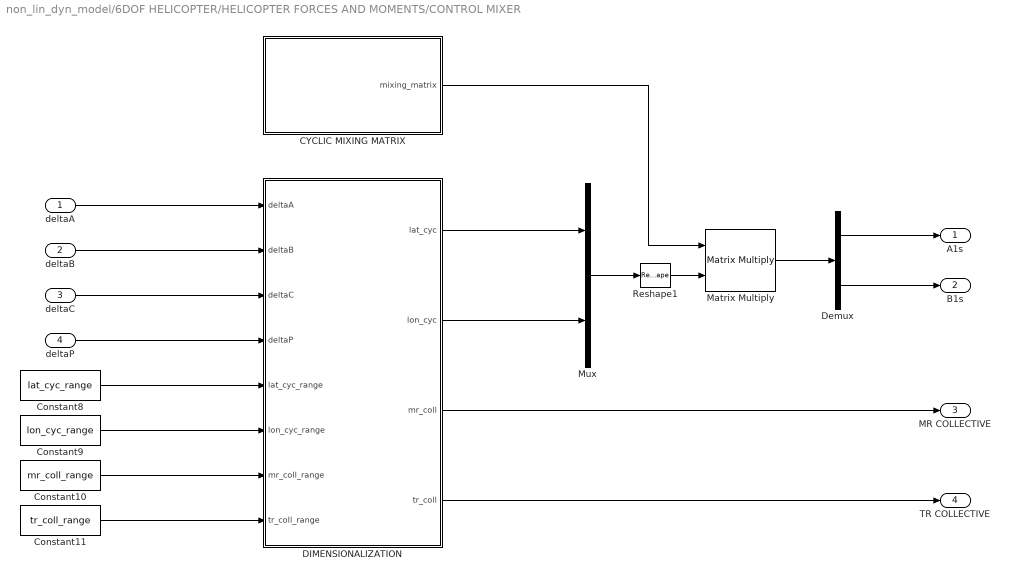
== system non_lin_dyn_model/6DOF HELICOPTER/HELICOPTER FORCES AND MOMENTS/CONTROL MIXER ==
  deltaA : Inport
  deltaB : Inport  Port=2
  deltaC : Inport  Port=3
  deltaP : Inport  Port=4
  CYCLIC MIXING MATRIX : MATLAB Function  TreatAsAtomicUnit=on
  Constant10 : Constant  Value=mr_coll_range
  Constant11 : Constant  Value=tr_coll_range
  Constant8 : Constant  Value=lat_cyc_range
  Constant9 : Constant  Value=lon_cyc_range
  DIMENSIONALIZATION : MATLAB Function  TreatAsAtomicUnit=on
  Demux : Demux  Outputs=2
  Matrix Multiply : Product  Multiplication=Matrix(*)
  Mux : Mux  Inputs=2
  Reshape1 : Reshape  OutputDimensionality=Column vector (2-D)
  A1s : Outport
  B1s : Outport  Port=2
  MR COLLECTIVE : Outport  Port=3
  TR COLLECTIVE : Outport  Port=4
  wires:
  Demux/2 -> B1s/1
  Matrix Multiply/1 -> Demux/1
  Mux/1 -> Reshape1/1
  Demux/1 -> A1s/1
  CYCLIC MIXING MATRIX/1(mixing_matrix) -> Matrix Multiply/1
  DIMENSIONALIZATION/1(lat_cyc) -> Mux/1
  DIMENSIONALIZATION/2(lon_cyc) -> Mux/2
  deltaP/1 -> DIMENSIONALIZATION/4(deltaP)
  deltaC/1 -> DIMENSIONALIZATION/3(deltaC)
  deltaB/1 -> DIMENSIONALIZATION/2(deltaB)
  deltaA/1 -> DIMENSIONALIZATION/1(deltaA)
  DIMENSIONALIZATION/3(mr_coll) -> MR COLLECTIVE/1
  DIMENSIONALIZATION/4(tr_coll) -> TR COLLECTIVE/1
  Constant8/1 -> DIMENSIONALIZATION/5(lat_cyc_range)
  Constant9/1 -> DIMENSIONALIZATION/6(lon_cyc_range)
  Constant10/1 -> DIMENSIONALIZATION/7(mr_coll_range)
  Constant11/1 -> DIMENSIONALIZATION/8(tr_coll_range)
  Reshape1/1 -> Matrix Multiply/2

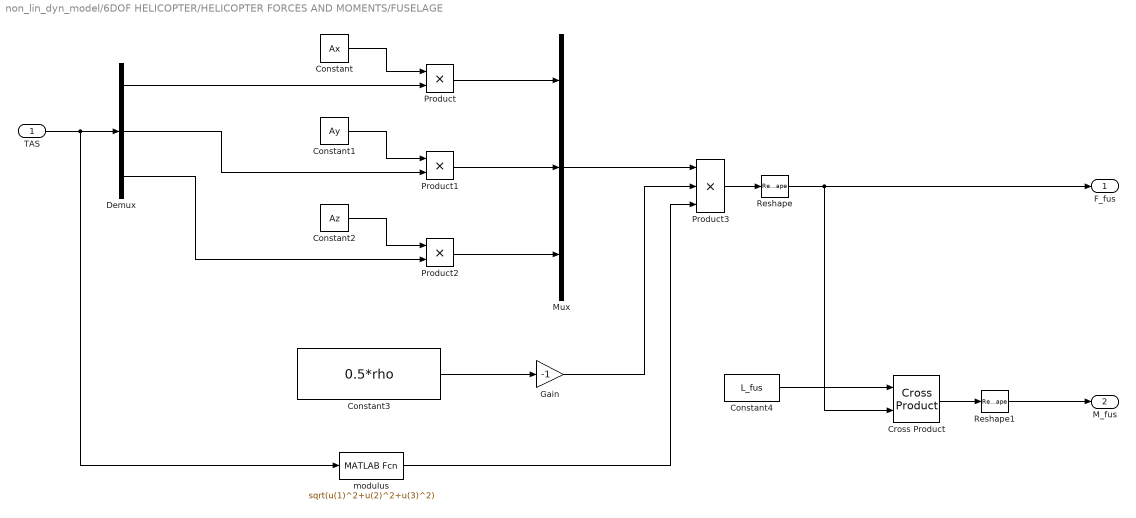
== system non_lin_dyn_model/6DOF HELICOPTER/HELICOPTER FORCES AND MOMENTS/FUSELAGE ==
  TAS : Inport
  Constant : Constant  Value=Ax
  Constant1 : Constant  Value=Ay
  Constant2 : Constant  Value=Az
  Constant3 : Constant  Value=0.5*rho
  Constant4 : Constant  Value=L_fus
  Cross Product : matrix_library/Cross Product
  Demux : Demux  Outputs=3
  Gain : Gain  Gain=-1
  Mux : Mux  Inputs=3
  Product : Product
  Product1 : Product
  Product2 : Product
  Product3 : Product  Inputs=3
  Reshape : Reshape  OutputDimensionality=Column vector (2-D)
  Reshape1 : Reshape  OutputDimensionality=Column vector (2-D)
  modulus : MATLABFcn  MATLABFcn=sqrt(u(1)^2+u(2)^2+u(3)^2)  OutputDimensions=1
  F_fus : Outport
  M_fus : Outport  Port=2
  wires:
  Demux/2 -> Product1/2
  modulus/1 -> Product3/3
  Product1/1 -> Mux/2
  Demux/1 -> Product/2
  Product/1 -> Mux/1
  Constant3/1 -> Gain/1
  Product2/1 -> Mux/3
  Product3/1 -> Reshape/1
  Reshape1/1 -> M_fus/1
  Constant/1 -> Product/1
  Demux/3 -> Product2/2
  TAS/1 -> modulus/1, Demux/1
  Constant1/1 -> Product1/1
  Constant2/1 -> Product2/1
  Constant4/1 -> Cross Product/1
  Reshape/1 -> F_fus/1, Cross Product/2
  Mux/1 -> Product3/1
  Cross Product/1 -> Reshape1/1
  Gain/1 -> Product3/2

== system non_lin_dyn_model/6DOF HELICOPTER/HELICOPTER FORCES AND MOMENTS/GRAVITY ==
  Tbe : Inport
  Constant : Constant  Value=[0;0;g]
  Gain : Gain  Gain=m
  Matrix Multiply : Product  Multiplication=Matrix(*)
  F_g : Outport
  wires:
  Matrix Multiply/1 -> F_g/1
  Constant/1 -> Gain/1
  Gain/1 -> Matrix Multiply/2
  Tbe/1 -> Matrix Multiply/1

== system non_lin_dyn_model/6DOF HELICOPTER/HELICOPTER FORCES AND MOMENTS/MAIN ROTOR ==
  TAS : Inport
  omega : Inport  Port=2
  A1s : Inport  Port=3
  B1s : Inport  Port=4
  theta0_mr : Inport  Port=5
  FLAPPING : Subsystem
  MAIN ROTOR FORCES : Subsystem
  F_mr : Outport
  M_mr : Outport  Port=2
  wires:
  MAIN ROTOR FORCES/2(M_mr) -> M_mr/1
  FLAPPING/1(a1s) -> MAIN ROTOR FORCES/3(a1s)
  A1s/1 -> FLAPPING/4(A1s)
  B1s/1 -> FLAPPING/5(B1s)
  TAS/1 -> FLAPPING/2(TAS), MAIN ROTOR FORCES/1(TAS)
  omega/1 -> FLAPPING/3(omega)
  FLAPPING/2(b1s) -> MAIN ROTOR FORCES/4(b1s)
  MAIN ROTOR FORCES/1(F_mr) -> F_mr/1
  theta0_mr/1 -> FLAPPING/1(theta0_mr), MAIN ROTOR FORCES/2(theta0_mr)
  MAIN ROTOR FORCES/3(inflow) -> FLAPPING/6(inflow)

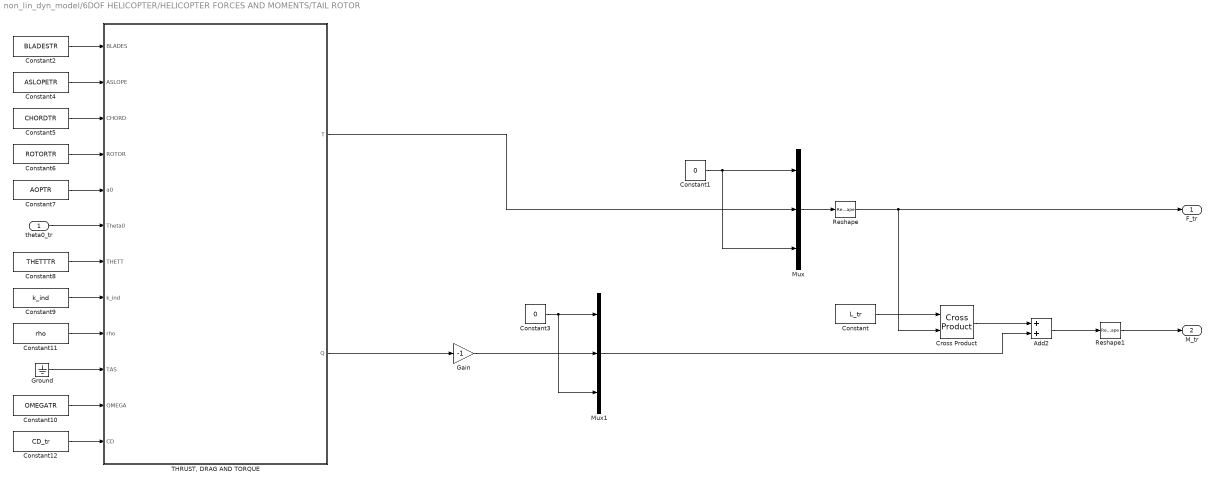
== system non_lin_dyn_model/6DOF HELICOPTER/HELICOPTER FORCES AND MOMENTS/TAIL ROTOR ==
  theta0_tr : Inport
  Add2 : Sum
  Constant : Constant  Value=L_tr
  Constant1 : Constant  Value=0
  Constant10 : Constant  Value=OMEGATR
  Constant11 : Constant  Value=rho
  Constant12 : Constant  Value=CD_tr
  Constant2 : Constant  Value=BLADESTR
  Constant3 : Constant  Value=0
  Constant4 : Constant  Value=ASLOPETR
  Constant5 : Constant  Value=CHORDTR
  Constant6 : Constant  Value=ROTORTR
  Constant7 : Constant  Value=AOPTR
  Constant8 : Constant  Value=THETTTR
  Constant9 : Constant  Value=k_ind
  Cross Product : matrix_library/Cross Product
  Gain : Gain  Gain=-1
  Ground : Ground
  Mux : Mux  Inputs=3
  Mux1 : Mux  Inputs=3
  Reshape : Reshape  OutputDimensionality=Column vector (2-D)
  Reshape1 : Reshape  OutputDimensionality=Column vector (2-D)
  "THRUST, DRAG AND TORQUE" : MATLAB Function  TreatAsAtomicUnit=on
  F_tr : Outport
  M_tr : Outport  Port=2
  wires:
  "THRUST, DRAG AND TORQUE"/1(T) -> Mux/2
  Constant3/1 -> Mux1/3, Mux1/1
  Mux1/1 -> Add2/2
  Mux/1 -> Reshape/1
  Constant1/1 -> Mux/3, Mux/1
  Gain/1 -> Mux1/2
  "THRUST, DRAG AND TORQUE"/2(Q) -> Gain/1
  Reshape/1 -> F_tr/1, Cross Product/2
  Constant/1 -> Cross Product/1
  Add2/1 -> Reshape1/1
  Cross Product/1 -> Add2/1
  Reshape1/1 -> M_tr/1
  Constant8/1 -> "THRUST, DRAG AND TORQUE"/7(THETT)
  Constant7/1 -> "THRUST, DRAG AND TORQUE"/5(a0)
  Constant6/1 -> "THRUST, DRAG AND TORQUE"/4(ROTOR)
  Constant9/1 -> "THRUST, DRAG AND TORQUE"/8(k_ind)
  Constant5/1 -> "THRUST, DRAG AND TORQUE"/3(CHORD)
  Constant10/1 -> "THRUST, DRAG AND TORQUE"/11(OMEGA)
  Constant2/1 -> "THRUST, DRAG AND TORQUE"/1(BLADES)
  theta0_tr/1 -> "THRUST, DRAG AND TORQUE"/6(Theta0)
  Constant11/1 -> "THRUST, DRAG AND TORQUE"/9(rho)
  Constant4/1 -> "THRUST, DRAG AND TORQUE"/2(ASLOPE)
  Ground/1 -> "THRUST, DRAG AND TORQUE"/10(TAS)
  Constant12/1 -> "THRUST, DRAG AND TORQUE"/12(CD)

== system non_lin_dyn_model/ATTITUDE CONTROLLER/ANGULAR RATE FEL CONTROLLER /filtered derivative ==
  x_sp : Inport
  Demux : Demux  Outputs=3
  Mux : Mux  Inputs=3
  Reshape2 : Reshape  OutputDimensionality=Column vector (2-D)
  filtered derivative : TransferFcn  Numerator=[1 0]  Denominator=[1/100 1]
  filtered derivative1 : TransferFcn  Numerator=[1 0]  Denominator=[1/100 1]
  filtered derivative2 : TransferFcn  Numerator=[1 0]  Denominator=[1/100 1]
  x_sp_dot : Outport
  wires:
  Demux/3 -> filtered derivative2/1
  Demux/1 -> filtered derivative/1
  Mux/1 -> Reshape2/1
  Demux/2 -> filtered derivative1/1
  filtered derivative1/1 -> Mux/2
  x_sp/1 -> Demux/1
  filtered derivative/1 -> Mux/1
  filtered derivative2/1 -> Mux/3
  Reshape2/1 -> x_sp_dot/1

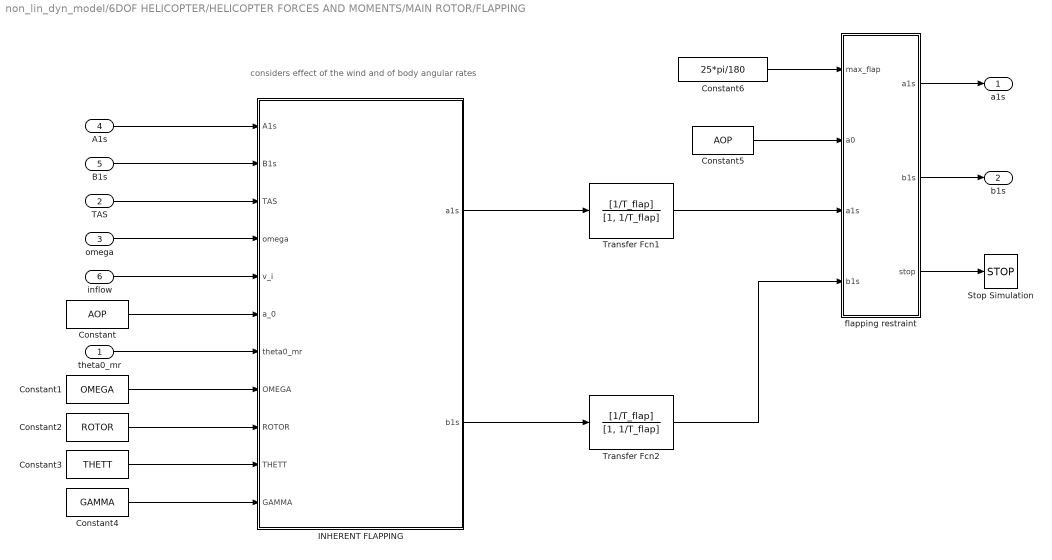
== system non_lin_dyn_model/6DOF HELICOPTER/HELICOPTER FORCES AND MOMENTS/MAIN ROTOR/FLAPPING ==
  note: considers effect of the wind and of body angular rates
  theta0_mr : Inport
  TAS : Inport  Port=2
  omega : Inport  Port=3
  A1s : Inport  Port=4
  B1s : Inport  Port=5
  inflow : Inport  Port=6
  Constant : Constant  Value=AOP
  Constant1 : Constant  Value=OMEGA
  Constant2 : Constant  Value=ROTOR
  Constant3 : Constant  Value=THETT
  Constant4 : Constant  Value=GAMMA
  Constant5 : Constant  Value=AOP
  Constant6 : Constant  Value=25*pi/180
  INHERENT FLAPPING : MATLAB Function  TreatAsAtomicUnit=on
  Stop Simulation : Stop
  Transfer Fcn1 : TransferFcn  Numerator=[1/T_flap]  Denominator=[1, 1/T_flap]
  Transfer Fcn2 : TransferFcn  Numerator=[1/T_flap]  Denominator=[1, 1/T_flap]
  flapping restraint : MATLAB Function  TreatAsAtomicUnit=on
  a1s : Outport
  b1s : Outport  Port=2
  wires:
  omega/1 -> INHERENT FLAPPING/4(omega)
  TAS/1 -> INHERENT FLAPPING/3(TAS)
  B1s/1 -> INHERENT FLAPPING/2(B1s)
  A1s/1 -> INHERENT FLAPPING/1(A1s)
  Constant6/1 -> flapping restraint/1(max_flap)
  Constant5/1 -> flapping restraint/2(a0)
  Transfer Fcn1/1 -> flapping restraint/3("a1s ")
  Transfer Fcn2/1 -> flapping restraint/4("b1s ")
  flapping restraint/1(a1s) -> a1s/1
  flapping restraint/2(b1s) -> b1s/1
  flapping restraint/3(stop) -> Stop Simulation/1
  Constant4/1 -> INHERENT FLAPPING/11(GAMMA)
  Constant3/1 -> INHERENT FLAPPING/10(THETT)
  Constant2/1 -> INHERENT FLAPPING/9(ROTOR)
  Constant1/1 -> INHERENT FLAPPING/8(OMEGA)
  theta0_mr/1 -> INHERENT FLAPPING/7(theta0_mr)
  inflow/1 -> INHERENT FLAPPING/5(v_i)
  Constant/1 -> INHERENT FLAPPING/6(a_0)
  INHERENT FLAPPING/2(b1s) -> Transfer Fcn2/1
  INHERENT FLAPPING/1(a1s) -> Transfer Fcn1/1

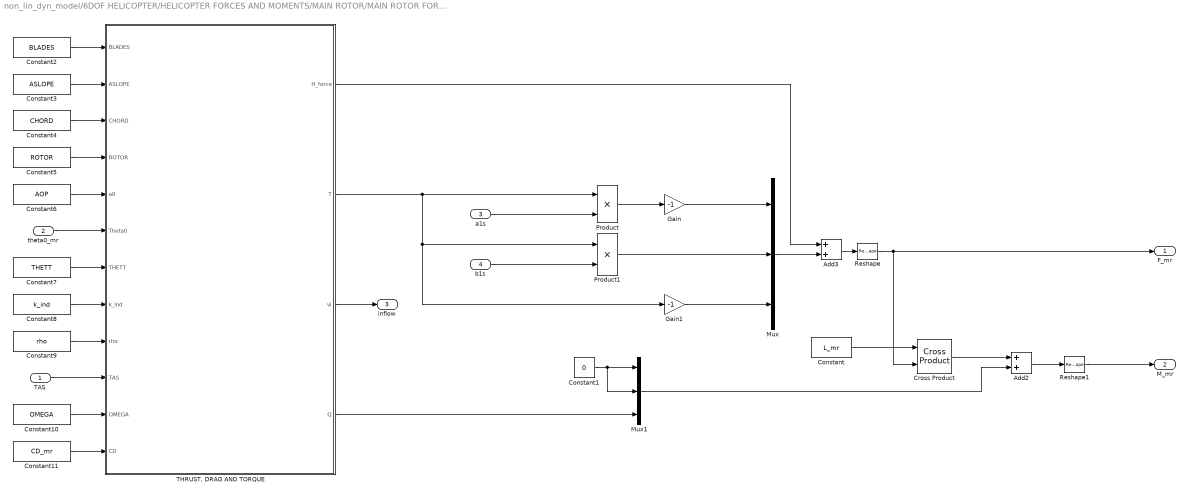
== system non_lin_dyn_model/6DOF HELICOPTER/HELICOPTER FORCES AND MOMENTS/MAIN ROTOR/MAIN ROTOR FORCES ==
  TAS : Inport
  theta0_mr : Inport  Port=2
  a1s : Inport  Port=3
  b1s : Inport  Port=4
  Add2 : Sum
  Add3 : Sum
  Constant : Constant  Value=L_mr
  Constant1 : Constant  Value=0
  Constant10 : Constant  Value=OMEGA
  Constant11 : Constant  Value=CD_mr
  Constant2 : Constant  Value=BLADES
  Constant3 : Constant  Value=ASLOPE
  Constant4 : Constant  Value=CHORD
  Constant5 : Constant  Value=ROTOR
  Constant6 : Constant  Value=AOP
  Constant7 : Constant  Value=THETT
  Constant8 : Constant  Value=k_ind
  Constant9 : Constant  Value=rho
  Cross Product : matrix_library/Cross Product
  Gain : Gain  Gain=-1
  Gain1 : Gain  Gain=-1
  Mux : Mux  Inputs=3
  Mux1 : Mux  Inputs=3
  Product : Product
  Product1 : Product
  Reshape : Reshape  OutputDimensionality=Column vector (2-D)
  Reshape1 : Reshape  OutputDimensionality=Column vector (2-D)
  "THRUST, DRAG AND TORQUE" : MATLAB Function  TreatAsAtomicUnit=on
  F_mr : Outport
  M_mr : Outport  Port=2
  inflow : Outport  Port=3
  wires:
  "THRUST, DRAG AND TORQUE"/1(H_force) -> Add3/1
  "THRUST, DRAG AND TORQUE"/2(T) -> Gain1/1, Product1/1, Product/1
  Product/1 -> Gain/1
  Cross Product/1 -> Add2/1
  a1s/1 -> Product/2
  Gain/1 -> Mux/1
  Add3/1 -> Reshape/1
  Mux/1 -> Add3/2
  Constant/1 -> Cross Product/1
  Add2/1 -> Reshape1/1
  Gain1/1 -> Mux/3
  b1s/1 -> Product1/2
  Product1/1 -> Mux/2
  "THRUST, DRAG AND TORQUE"/4(Q) -> Mux1/3
  Constant1/1 -> Mux1/2, Mux1/1
  Mux1/1 -> Add2/2
  Reshape/1 -> F_mr/1, Cross Product/2
  Reshape1/1 -> M_mr/1
  "THRUST, DRAG AND TORQUE"/3(vi) -> inflow/1
  Constant9/1 -> "THRUST, DRAG AND TORQUE"/9(rho)
  Constant10/1 -> "THRUST, DRAG AND TORQUE"/11(OMEGA)
  Constant8/1 -> "THRUST, DRAG AND TORQUE"/8(k_ind)
  Constant7/1 -> "THRUST, DRAG AND TORQUE"/7(THETT)
  Constant6/1 -> "THRUST, DRAG AND TORQUE"/5(a0)
  Constant5/1 -> "THRUST, DRAG AND TORQUE"/4(ROTOR)
  Constant4/1 -> "THRUST, DRAG AND TORQUE"/3(CHORD)
  Constant3/1 -> "THRUST, DRAG AND TORQUE"/2(ASLOPE)
  Constant2/1 -> "THRUST, DRAG AND TORQUE"/1(BLADES)
  Constant11/1 -> "THRUST, DRAG AND TORQUE"/12(CD)
  theta0_mr/1 -> "THRUST, DRAG AND TORQUE"/6(Theta0)
  TAS/1 -> "THRUST, DRAG AND TORQUE"/10(TAS)

== matlab function non_lin_dyn_model/6DOF HELICOPTER/HELICOPTER FORCES AND MOMENTS/MAIN ROTOR/MAIN ROTOR FORCES/THRUST, DRAG AND TORQUE ==
  data: H_force output; BLADES input; T output; vi output; ASLOPE input; CHORD input; ROTOR input; a0 input; Theta0 input; THETT input; k_ind input; rho input; TAS input; OMEGA input; Q output; CD input
function [H_force,T,vi,Q] = fcn(BLADES,ASLOPE,CHORD,ROTOR,a0,Theta0,THETT,k_ind,rho,TAS,OMEGA,CD)

%% preliminary calculations
A = pi*ROTOR^2; % area of rotor disc 
sigma = BLADES*CHORD/(pi*ROTOR); % solidity of rotor 
uH = TAS(1);
vH = TAS(2);
wH = TAS(3);
beta_w = atan2(vH,uH); % sideslip angle 
Mu = sqrt(uH^2+vH^2)/(OMEGA*ROTOR); % advance ratio

%% thrust calculation
lambda = fzero(@(x) x-wH/(OMEGA*ROTOR)+0.5*((0.5*BLADES*rho*ASLOPE*CHORD*ROTOR*(OMEGA*ROTOR)^2*(x/2+Theta0*(1/3+Mu^2/2)+THETT*(1/4+Mu^2/4)))/(rho*A*(OMEGA*ROTOR)^2))/sqrt(Mu^2+x^2), -0.1);
vi = wH-lambda*OMEGA*ROTOR;
T = (0.5*BLADES*rho*ASLOPE*CHORD*ROTOR*(OMEGA*ROTOR)^2*(lambda/2+Theta0*(1/3+Mu^2/2)+THETT*(1/4+Mu^2/4)));
CT = T/(rho*A*(OMEGA*ROTOR)^2);
alpha_mean = 6*CT/ASLOPE/sigma;
delta = CD(1)+CD(2)*alpha_mean+CD(3)*alpha_mean^2;

%% forces and moments in the hub-wind frame

H_w = BLADES/2*rho*ASLOPE*CHORD*ROTOR*(OMEGA*ROTOR)^2*(delta*Mu/(2*ASLOPE)-1/4*Theta0*(2*lambda*Mu) ...
      -THETT/4*(Mu*lambda)+Mu/4*a0^2);

Q = k_ind*BLADES/2*rho*ASLOPE*CHORD*ROTOR^2*(OMEGA*ROTOR)^2*(delta/k_ind/(4*ASLOPE)*(1+Mu^2)-Theta0*(lambda/3) ...
    -THETT*lambda/4-1/2*lambda^2);

%% rotation from hub_wind to hub-body axis:
H_force = [-H_w*cos(beta_w);
           -H_w*sin(beta_w);
                 0         ];

== matlab function non_lin_dyn_model/6DOF HELICOPTER/HELICOPTER FORCES AND MOMENTS/TAIL ROTOR/THRUST, DRAG AND TORQUE ==
  data: BLADES input; T output; ASLOPE input; CHORD input; ROTOR input; a0 input; Theta0 input; THETT input; k_ind input; rho input; TAS input; OMEGA input; Q output; CD input
function [T,Q] = fcn(BLADES,ASLOPE,CHORD,ROTOR,a0,Theta0,THETT,k_ind,rho,TAS,OMEGA,CD)

%% preliminary calculations
A = pi*ROTOR^2; % area of rotor disc 
sigma = BLADES*CHORD/(pi*ROTOR); % solidity of rotor 
uH = 0;
vH = 0;
wH = 0;
beta_w = atan2(vH,uH); % sideslip angle 
Mu = sqrt(uH^2+vH^2)/(OMEGA*ROTOR); % advance ratio

%% thrust calculation
lambda = fzero(@(x) x-wH/(OMEGA*ROTOR)+0.5*((0.5*BLADES*rho*ASLOPE*CHORD*ROTOR*(OMEGA*ROTOR)^2*(x/2+Theta0*(1/3+Mu^2/2)+ ...
    +THETT*(1/4+Mu^2/4)))/(rho*A*(OMEGA*ROTOR)^2))/sqrt(Mu^2+x^2), -0.1);
vi = wH-lambda*OMEGA*ROTOR;
T = (0.5*BLADES*rho*ASLOPE*CHORD*ROTOR*(OMEGA*ROTOR)^2*(lambda/2+Theta0*(1/3+Mu^2/2)+ ...
    +THETT*(1/4+Mu^2/4)));
CT = T/(rho*A*(OMEGA*ROTOR)^2);
alpha_mean = 6*CT/ASLOPE/sigma;
delta = CD(1)+CD(2)*alpha_mean+CD(3)*alpha_mean^2;

%% forces and moments in the hub-wind frame

H_w = BLADES/2*rho*ASLOPE*CHORD*ROTOR*(OMEGA*ROTOR)^2*(delta*Mu/(2*ASLOPE)-1/4*Theta0*(2*lambda*Mu) ...
      -THETT/4*(Mu*lambda)+Mu/4*a0^2);

Q = k_ind*BLADES/2*rho*ASLOPE*CHORD*ROTOR^2*(OMEGA*ROTOR)^2*(delta/k_ind/(4*ASLOPE)*(1+Mu^2)-Theta0*(lambda/3) ...
    -THETT*lambda/4-1/2*lambda^2);

%% rotation from hub_wind to hub-body axis:
H_force = [-H_w*cos(beta_w);
           -H_w*sin(beta_w);
                 0         ];

== matlab function non_lin_dyn_model/ATTITUDE CONTROLLER/NEURAL NETWORK /activation functions ==
  data: X_bar input; x0 input; sigma input; mu output
function mu = fcn(X_bar, x0, sigma)

mu = x0*0;
for i=1:length(mu)
    mu(i,1) = exp(-((X_bar-x0(i))'*(X_bar-x0(i)))/(2*sigma(i)^2));
end

== matlab function non_lin_dyn_model/ATTITUDE CONTROLLER/NEURAL NETWORK /input normalization ==
  data: X input; Xbar output
function Xbar = fcn(X)

% X = [ phidot,thetadot,psidot, phi,theta,psi, deltaA,deltaB,deltaP ]
% controls are already normalized

max_rate  = 2;      % expected max angular rate [rad/s]
max_angle = pi/2;   % expected max attitude angle [rad]

Xbar = [  X(1)/max_rate ;
          X(2)/max_rate ;
          X(3)/max_rate ;
          X(4)/max_angle;
          X(5)/max_angle;
          X(6)/max_angle;
          X(7)          ;
          X(8)          ;
          X(9)          ];

== matlab function non_lin_dyn_model/ATTITUDE CONTROLLER/NEURAL NETWORK /update rule ==
  data: eta input; s input; mu input; W output; W0 input; ST input
function W = fcn(eta,s,mu,W0,ST)

sigma = 0.01;
dWdt = eta*(mu*s'-sigma*W0);
W = W0+dWdt*ST;

== matlab function non_lin_dyn_model/POSITION CONTROLLER /ACCELERATION AND YAW TO ATTITUDE/MATLAB Function ==
  data: phi_sp output; Asp input; theta_sp output; g0 input; psi input
function [phi_sp,theta_sp] = fcn(Asp,g0,psi)
% step 1: normalization
I_e_cmd_z = (Asp-[0 0 g0]')/(norm(Asp-[0 0 g0]'));
% step 2: rotation around local z
K_e_cmd_z = [cos(psi) sin(psi) 0; -sin(psi) cos(psi) 0; 0       0       1]*I_e_cmd_z;
% step 3: calculation of pitch and roll angles
theta_sp = atan(K_e_cmd_z(1)/K_e_cmd_z(3));
phi_sp = atan(-1/cos(theta_sp)*(K_e_cmd_z(2)*K_e_cmd_z(3))/(K_e_cmd_z(1)^2+K_e_cmd_z(3)^2));

== matlab function non_lin_dyn_model/Wind disturbance ==
  data: t input; W output; wind input
function W = fcn(t,wind)

Wxy = 5;
Wz  = 0;
T   = 8;
if wind ==1
    W=[ Wxy*sin((1/T)*2*pi*t+pi/4);
        Wxy*sin((1/T)*2*pi*t+pi/4);
         Wz*sin((1/T)*2*pi*t+pi/4)];
else
    W=[ 0;
        0;
        0];
end

== matlab function non_lin_dyn_model/POSITION CONTROLLER /VERTICAL CHANNELL CONTROLLER/MATLAB Function ==
  data: Asp_z input; delta_vert output; g0 input
function delta_vert = fcn(Asp_z,g0)

delta_vert = -Asp_z/g0; % basically the load factor

== matlab function non_lin_dyn_model/POSITION CONTROLLER /reference trajectory ==
  data: Psi_sp output; t input; X_sp output; Xe_0 input; Xe input
function [Psi_sp,X_sp] = fcn(t,Xe_0,Xe)

R = 8;
T = 30;
X_sp=[ R*cos(2*pi/T*t) - R + Xe_0(1) ;
       R*sin(2*pi/T*t)     + Xe_0(2) ;
                   Xe(3)            ];
%Psi_sp  = 2*pi/T*t + pi/2;
%Psi_sp = mod(2*pi/T*t + pi/2 + pi, 2*pi) - pi;
Psi_sp = pi/2*0;
